simulink model "test_feedback_linearization_corrected_function"  (R2022b)
settings: Solver=VariableStepAuto  StartTime=0.0  StopTime=0.5  RelTol=1e-3
values from neighbouring files (symbols this model uses):
  I_m = [params.permanent.J/params.physical.mu0*params.permanent.l(1) ... (first row only)    [pole_placement.m]
  K_tst = place(A_n,B_n,poles)    [pole_placement.m]
  x0 = x_lp+[0.01,0,0.02, zeros(1,9)]'    [main.m]
  x_lp = [0,0,0.047,zeros(1,9)]'    [main.m]
settings Model: Creator=pal12  LastModifiedBy=pal12

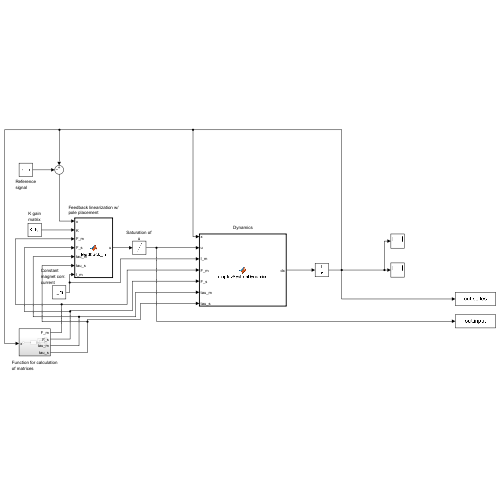
[thumbnail: Simulink's stored preview of the top-level diagram]
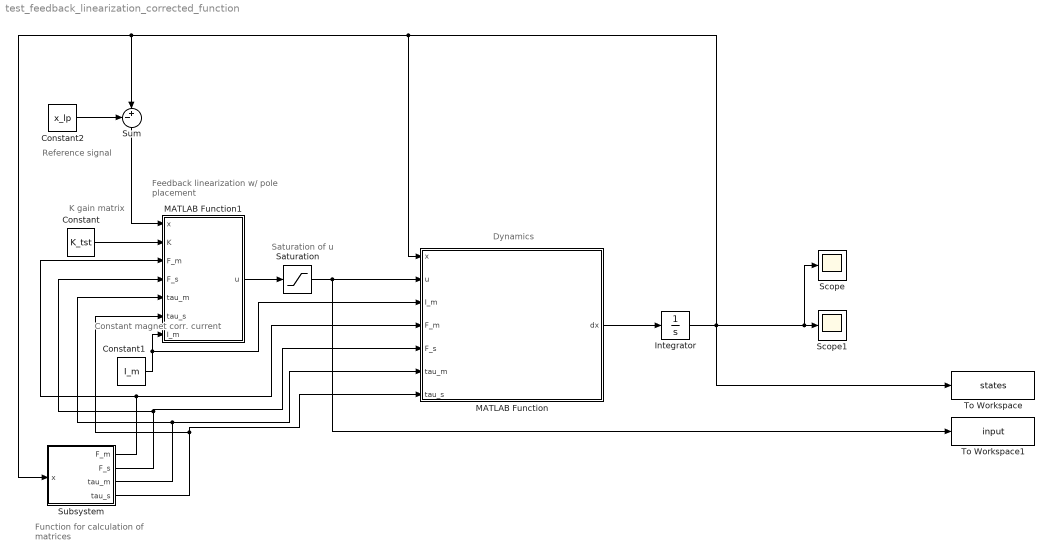
== system test_feedback_linearization_corrected_function ==
  note: Dynamics
  note: Saturation of
      | u
  note: Constant
      | magnet corr.
      | current
  note: K gain
      | matrix
  note: Reference
      | signal
  note: Function for calculation
      | of matrices
  note: Feedback linearization w/
      | pole placement
  Constant : Constant  Value=K_tst
  Constant1 : Constant  Value=I_m
  Constant2 : Constant  Value=x_lp
  Integrator : Integrator  InitialCondition=x0
  MATLAB Function : MATLAB Function  TreatAsAtomicUnit=on
  MATLAB Function1 : MATLAB Function  TreatAsAtomicUnit=on
  Saturation : Saturate  UpperLimit=200  LowerLimit=-200
  Scope : Scope
  Scope1 : Scope
  Subsystem : Subsystem
  Sum : Sum  Inputs=-+|
  To Workspace : ToWorkspace  VariableName=states  SampleTime=-1
      settings: Save2DSignal=2-D array (concatenate along first dimension)
  To Workspace1 : ToWorkspace  VariableName=input  SampleTime=-1
  wires:
  MATLAB Function/1(dx) -> Integrator/1
  Constant/1 -> MATLAB Function1/2(K)
  Constant1/1 -> MATLAB Function/3(I_m), MATLAB Function1/7(I_m)
  Integrator/1 -> MATLAB Function/1(x), Subsystem/1(x), Sum/2, Scope/1, Scope1/1, To Workspace/1
  MATLAB Function1/1(u) -> Saturation/1
  Saturation/1 -> MATLAB Function/2(u), To Workspace1/1
  Sum/1 -> MATLAB Function1/1(x)
  Constant2/1 -> Sum/1
  Subsystem/1(F_m) -> MATLAB Function1/3(F_m), MATLAB Function/4(F_m)
  Subsystem/2(F_s) -> MATLAB Function/5(F_s), MATLAB Function1/4(F_s)
  Subsystem/3(tau_m) -> MATLAB Function/6(tau_m), MATLAB Function1/5(tau_m)
  Subsystem/4(tau_s) -> MATLAB Function/7(tau_s), MATLAB Function1/6(tau_s)

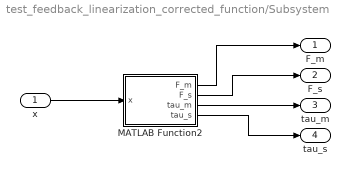
== system test_feedback_linearization_corrected_function/Subsystem ==
  x : Inport
  MATLAB Function2 : MATLAB Function  TreatAsAtomicUnit=on
  F_m : Outport
  F_s : Outport  Port=2
  tau_m : Outport  Port=3
  tau_s : Outport  Port=4
  wires:
  MATLAB Function2/2(F_s) -> F_s/1
  MATLAB Function2/1(F_m) -> F_m/1
  x/1 -> MATLAB Function2/1(x)
  MATLAB Function2/3(tau_m) -> tau_m/1
  MATLAB Function2/4(tau_s) -> tau_s/1

== matlab function test_feedback_linearization_corrected_function/MATLAB Function1 ==
  data: x input; K input; u output; params parameter; F_m input; F_s input; tau_m input; tau_s input; I_m input
function u = feedback_ln(x, K, params, F_m, F_s, tau_m, tau_s, I_m)

    g = [
    params.magnet.m*eye(3), zeros(3);
    zeros(3), diag(params.magnet.I)
    ];

    h = [zeros(3,1); cross(x(10:12),diag(params.magnet.I)*x(10:12))]-[zeros(2,1);params.physical.g;zeros(3,1)];

    Fs = [F_s;tau_s];
    Fm = [F_m;tau_m];

    u = Fs\(h-Fm*I_m-g*K*x);
    %u = -K*x([1:5,7:11]);%linearization

== matlab function test_feedback_linearization_corrected_function/MATLAB Function ==
  data: x input; u input; I_m input; dx output; params parameter; F_m input; F_s input; tau_m input; tau_s input
function dx = maglevSystemDynamics(x,u,I_m,params,F_m,F_s,tau_m,tau_s)
    %{
    Computes the derivative of the state for a magnetic levitation system.
    - x: current state
    - u: control input
    - params: system parameters
    %}

    F = F_m*I_m+F_s*u;
    tau = tau_m*I_m+tau_s*u;
    
    % Setting up system matrices
    A = [
        zeros(6), eye(6);
        zeros(6), zeros(6)
        ];

    B = [
        zeros(6);
        eye(6)
        ];
    
    % Mass and inertia properties of the magnet
    M = [
        params.magnet.m*eye(3), zeros(3);
        zeros(3), diag(params.magnet.I)
        ];
    
    % Computing the nonlinear function f(x,u)
    f = M\([F;tau]-[zeros(3,1); cross(x(10:12),diag(params.magnet.I)*x(10:12))])-[zeros(2,1);params.physical.g;zeros(3,1)];
    
    dx = A*x+B*f;
end

== matlab function test_feedback_linearization_corrected_function/Subsystem/MATLAB Function2 ==
  data: F_m output; F_s output; tau_m output; tau_s output; x input; params parameter
function [F_m,F_s,tau_m,tau_s] = fcn(x,params)
[F_m,F_s,tau_m,tau_s] = force(x,params);
